simulink model "triggered"  (R2018a)
settings: Solver=ode45  StartTime=0.0  StopTime=10.0  RelTol=1e-3  EnableMultiTasking=on
settings Model: Creator=nicholas  LastModifiedBy=bneiswan
settings DataIOCC: LimitDataPoints=on  SaveFormat=Array  SignalLoggingName=sigsOut
settings OptimizationCC: ExpressionDepthLimit=2147483647  InitFltsAndDblsToZero=on  LifeSpan=inf
settings DebuggingCC: SaveWithParameterizedLinksMsg=none  UnderspecifiedInitializationDetection=Classic  MergeDetectMultiDrivingBlocksExec=none  CheckExecutionContextPreStartOutputMsg=on  CheckExecutionContextRuntimeOutputMsg=on  SignalResolutionControl=TryResolveAllWithWarning  MultiTaskDSMMsg=warning  MultiTaskCondExecSysMsg=none  ParameterPrecisionLossMsg=none  FcnCallInpInsideContextMsg=warning  AllowSymbolicDim=off  StateNameClashWarn=warning  SFUnexpectedBacktrackingDiag=warning  SFNoUnconditionalDefaultTransitionDiag=warning  SFExecutionAtInitializationDiag=none
settings HardwareCC: ProdBitPerPointer=32  ProdBitPerSizeT=32  ProdBitPerPtrDiffT=32  ProdLargestAtomicFloat=None  ProdIntDivRoundTo=Undefined  ProdEndianess=Unspecified  ProdWordSize=32  ProdHWDeviceType=32-bit Generic  TargetUnknown=on
settings ModelReferenceCC: PropagateSignalLabelsOutOfModel=off
settings CodeAppCC: StateflowObjectComments=on
settings GRTTargetCC: TargetFcnLib=ansi_tfl_tmw.mat  TargetLangStandard=C89/C90 (ANSI)  GeneratePreprocessorConditionals=Disable all  CombineOutputUpdateFcns=off  GRTInterface=on
settings ConfigComp: CovMetricSettings=dw  CovHtmlReporting=on  CovSaveCumulativeToWorkspaceVar=on  CovSaveSingleToWorkspaceVar=on  CovExternalEMLEnable=off  CovSFcnEnable=off

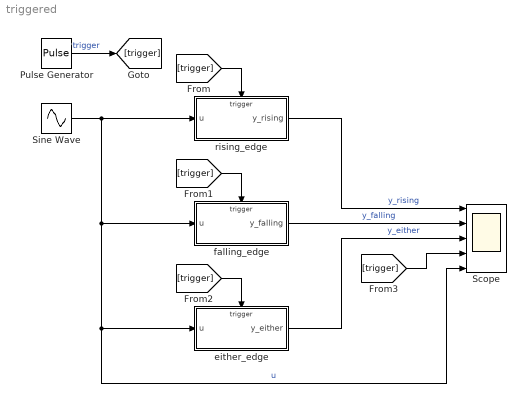
== system triggered ==
  Pulse Generator : DiscretePulseGenerator  PulseType=Time based  Amplitude=4  PulseWidth=50
  Scope : Scope  NumInputPorts=5
  Sine Wave : Sin  Amplitude=4  SampleTime=0
  either_edge : Subsystem  TreatAsAtomicUnit=on
  falling_edge : Subsystem  TreatAsAtomicUnit=on
  rising_edge : Subsystem  TreatAsAtomicUnit=on
  wires:
  falling_edge/1(y_falling) -> Scope/2  "y_falling"
  rising_edge/1(y_rising) -> Scope/1  "y_rising"
  either_edge/1(y_either) -> Scope/3  "y_either"
  Sine Wave/1 -> rising_edge/1(u), falling_edge/1(u), Scope/5, either_edge/1(u)  "u"
  Pulse Generator/1 -> [trigger]  "trigger"
  [trigger] -> rising_edge/Trigger
  [trigger] -> falling_edge/Trigger
  [trigger] -> either_edge/Trigger
  [trigger] -> Scope/4

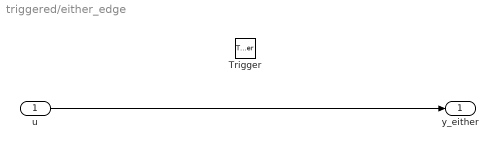
== system triggered/either_edge ==
  u : Inport
  Trigger : TriggerPort  TriggerType=either  VariantControl=Variant
  y_either : Outport
  wires:
  u/1 -> y_either/1

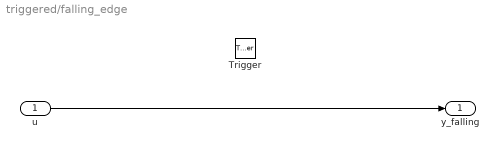
== system triggered/falling_edge ==
  u : Inport
  Trigger : TriggerPort  TriggerType=falling  VariantControl=Variant
  y_falling : Outport
  wires:
  u/1 -> y_falling/1

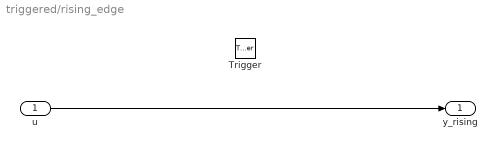
== system triggered/rising_edge ==
  u : Inport
  Trigger : TriggerPort  VariantControl=Variant
  y_rising : Outport
  wires:
  u/1 -> y_rising/1
